simulink model "lab3"  (R2023a)
settings: Solver=VariableStepAuto  StartTime=0.0  StopTime=10.0  RelTol=1e-3
settings Model: Creator=bkate  LastModifiedBy=bkate

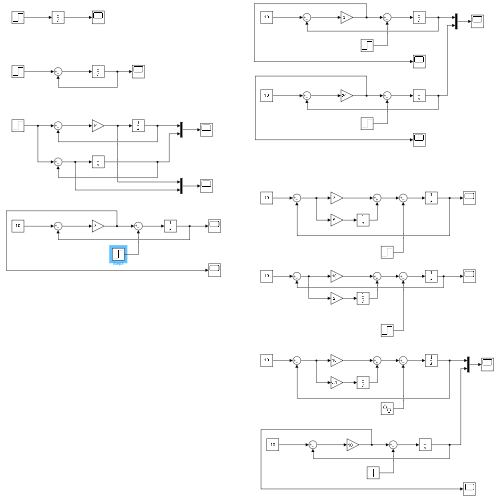
[thumbnail: Simulink's stored preview of the top-level diagram]
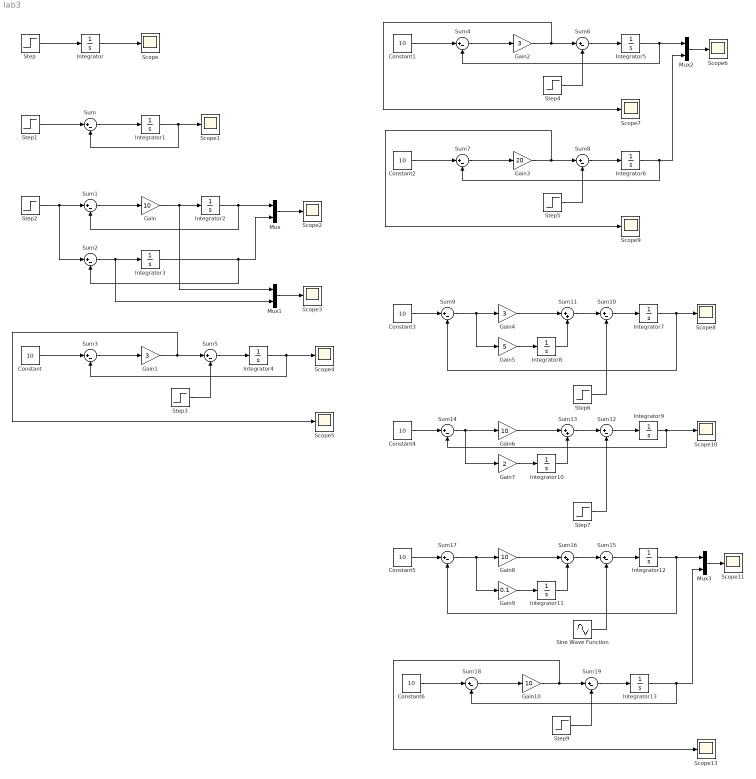
== system lab3 ==
  Constant{,1..6} (7 alike) : Constant  Value=10
  Gain{,6,8,10} (4 alike) : Gain  Gain=10
  Gain1 : Gain  Gain=3
  Gain2 : Gain  Gain=3
  Gain3 : Gain  Gain=20
  Gain4 : Gain  Gain=3
  Gain5 : Gain  Gain=5
  Gain7 : Gain  Gain=2
  Gain9 : Gain  Gain=0.1
  Integrator{,1..13} (14 alike) : Integrator
  Mux{,1..3} (4 alike) : Mux  Inputs=2
  Scope{,1..11,13} (13 alike) : Scope
  Sine Wave Function : Sin  Amplitude=4  Frequency=2  SampleTime=0
  Step : Step  SampleTime=0
  Step1 : Step  SampleTime=0
  Step2 : Step  SampleTime=0
  Step{3..7,9} (6 alike) : Step  Time=5  SampleTime=0
  Sum{,1..10,12,14..15,17..19} (17 alike) : Sum  Inputs=|+-
  Sum11 : Sum  Inputs=|++
  Sum13 : Sum  Inputs=|++
  Sum16 : Sum  Inputs=|++
  wires:
  Step/1 -> Integrator/1
  Integrator/1 -> Scope/1
  Integrator1/1 -> Sum/2, Scope1/1
  Step1/1 -> Sum/1
  Sum/1 -> Integrator1/1
  Sum1/1 -> Gain/1
  Integrator2/1 -> Mux/1, Sum1/2
  Step2/1 -> Sum2/1, Sum1/1
  Gain/1 -> Mux1/1, Integrator2/1
  Sum2/1 -> Mux1/2, Integrator3/1
  Integrator3/1 -> Mux/2, Sum2/2
  Mux/1 -> Scope2/1
  Mux1/1 -> Scope3/1
  Integrator4/1 -> Scope4/1, Sum3/2
  Constant/1 -> Sum3/1
  Sum3/1 -> Gain1/1
  Sum5/1 -> Integrator4/1
  Step3/1 -> Sum5/2
  Gain1/1 -> Sum5/1, Scope5/1
  Constant1/1 -> Sum4/1
  Integrator5/1 -> Mux2/1, Sum4/2
  Sum6/1 -> Integrator5/1
  Sum4/1 -> Gain2/1
  Gain2/1 -> Sum6/1, Scope7/1
  Step4/1 -> Sum6/2
  Step5/1 -> Sum8/2
  Gain3/1 -> Sum8/1, Scope9/1
  Sum7/1 -> Gain3/1
  Sum8/1 -> Integrator6/1
  Integrator6/1 -> Mux2/2, Sum7/2
  Constant2/1 -> Sum7/1
  Mux2/1 -> Scope6/1
  Integrator7/1 -> Scope8/1, Sum9/2
  Constant3/1 -> Sum9/1
  Sum10/1 -> Integrator7/1
  Sum9/1 -> Gain5/1, Gain4/1
  Step6/1 -> Sum10/2
  Gain4/1 -> Sum11/1
  Sum11/1 -> Sum10/1
  Gain5/1 -> Integrator8/1
  Integrator8/1 -> Sum11/2
  Sum13/1 -> Sum12/1
  Gain7/1 -> Integrator10/1
  Gain6/1 -> Sum13/1
  Sum14/1 -> Gain7/1, Gain6/1
  Constant4/1 -> Sum14/1
  Sum12/1 -> Integrator9/1
  Step7/1 -> Sum12/2
  Integrator10/1 -> Sum13/2
  Integrator9/1 -> Scope10/1, Sum14/2
  Integrator12/1 -> Mux3/1, Sum17/2
  Sum15/1 -> Integrator12/1
  Constant5/1 -> Sum17/1
  Integrator11/1 -> Sum16/2
  Gain8/1 -> Sum16/1
  Sum17/1 -> Gain9/1, Gain8/1
  Gain9/1 -> Integrator11/1
  Sum16/1 -> Sum15/1
  Constant6/1 -> Sum18/1
  Integrator13/1 -> Mux3/2, Sum18/2
  Sum19/1 -> Integrator13/1
  Sum18/1 -> Gain10/1
  Gain10/1 -> Sum19/1, Scope13/1
  Step9/1 -> Sum19/2
  Sine Wave Function/1 -> Sum15/2
  Mux3/1 -> Scope11/1
